simulink model "Evaluate_inertia_and_damping"  (R2016b)
settings: Solver=ode1  StartTime=0.0  StopTime=pre_time + s_t  FixedStep=T_sample  MinStep=1e-4  RelTol=1e-3
undefined symbols (not defined in the file): Activator, pre_time, selector
libraries: qbmove_library x2, QB_pacer_lib x1
settings Model: Creator=Franco  LastModifiedBy=Franco
settings DataIOCC: LimitDataPoints=on  SaveFormat=Array  SignalLoggingSaveFormat=ModelDataLogs
settings OptimizationCC: ExpressionDepthLimit=2147483647  EfficientMapNaN2IntZero=off  LifeSpan=inf
settings DebuggingCC: UnderspecifiedInitializationDetection=Classic  MergeDetectMultiDrivingBlocksExec=none  SolverPrmCheckMsg=warning  FcnCallInpInsideContextMsg=warning  AllowSymbolicDim=off  StateNameClashWarn=warning  SFUnexpectedBacktrackingDiag=warning  SFNoUnconditionalDefaultTransitionDiag=warning  SFExecutionAtInitializationDiag=none
settings HardwareCC: ProdBitPerPointer=32  ProdBitPerSizeT=32  ProdBitPerPtrDiffT=32  ProdLargestAtomicFloat=None  ProdIntDivRoundTo=Undefined  ProdEndianess=Unspecified  ProdWordSize=32  ProdHWDeviceType=32-bit Generic  TargetBitPerPointer=64  TargetBitPerSizeT=64  TargetBitPerPtrDiffT=64  TargetLongLongMode=on  TargetIntDivRoundTo=Zero  TargetEndianess=LittleEndian  TargetWordSize=64  TargetHWDeviceType=MATLAB Host  ProdEqTarget=off
settings ModelReferenceCC: PropagateSignalLabelsOutOfModel=off
settings CodeAppCC: MaxIdLength=128
settings GRTTargetCC: TargetLangStandard=C89/C90 (ANSI)  GeneratePreprocessorConditionals=Disable all  CombineOutputUpdateFcns=off  GRTInterface=on
settings ConfigComp: CovMetricSettings=dw  CovHtmlReporting=on  CovSaveCumulativeToWorkspaceVar=on  CovSaveSingleToWorkspaceVar=on  CovExternalEMLEnable=off  CovSFcnEnable=off
settings ConfigurationSet: Description=SimMechanics 2G

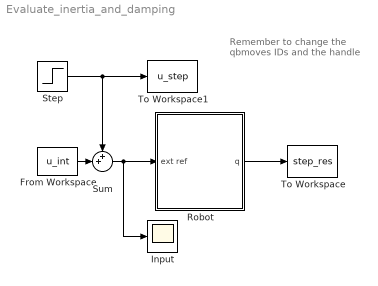
== system Evaluate_inertia_and_damping ==
  note: Remember to change the qbmoves IDs and the handle
  From Workspace : FromWorkspace  VariableName=u_int  SampleTime=0  OutputAfterFinalValue=Setting to zero
  Input : Scope
  Robot : Subsystem
  Step : Step  Time=pre_time  After=selector  SampleTime=0
  Sum : Sum  Inputs=++|
  To Workspace : ToWorkspace  VariableName=step_res  SaveFormat=Structure With Time  SampleTime=-1
  To Workspace1 : ToWorkspace  VariableName=u_step  SaveFormat=Structure With Time  SampleTime=-1
  wires:
  From Workspace/1 -> Sum/2
  Sum/1 -> Robot/1("ext ref "), Input/1
  Step/1 -> Sum/1, To Workspace1/1
  Robot/1(q) -> To Workspace/1

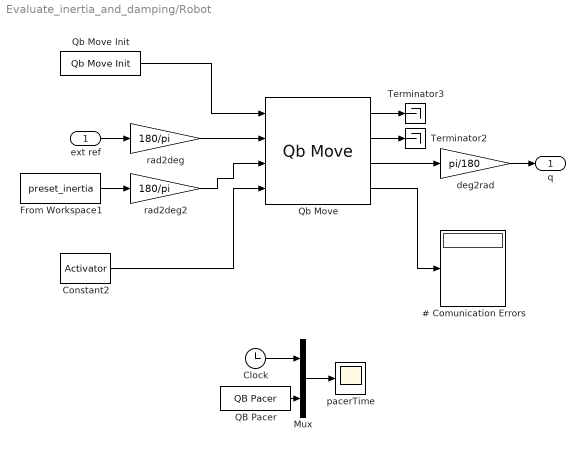
== system Evaluate_inertia_and_damping/Robot ==
  "ext ref " : Inport
  # Comunication Errors : Display
  Clock : Clock
  Constant2 : Constant  Value=Activator
  From Workspace1 : FromWorkspace  VariableName=preset_inertia  SampleTime=0  OutputAfterFinalValue=Setting to zero
  Mux : Mux  Inputs=2
  QB Pacer : QB_pacer_lib/QB Pacer  simTimePerRealTime=1
  Qb Move : qbmove_library/Qb Move  ID=[1 2 3 4 5 6]  ACTIVE_COMM_DIRECTIONS=Both  CONTROL_MODE=Equilibrium Position and Stiffness Preset  DAISY_CHAINING=off  MAX_ANG=0  SW_LIMIT=inf  OFFSET=0  ACTIVATE=off  WDT=0.0  UNIT=Degrees
  Qb Move Init : qbmove_library/Qb Move Init  NUMBER_OF_COM='COM7'  BAUD_RATE_COM=2000000
  Terminator2 : Terminator
  Terminator3 : Terminator
  deg2rad : Gain  Gain=pi/180
  pacerTime : Scope
  rad2deg : Gain  Gain=180/pi
  rad2deg2 : Gain  Gain=180/pi
  q : Outport
  wires:
  deg2rad/1 -> q/1
  "ext ref "/1 -> rad2deg/1
  From Workspace1/1 -> rad2deg2/1
  QB Pacer/1 -> Mux/2
  Clock/1 -> Mux/1
  Qb Move Init/1 -> Qb Move/1
  Mux/1 -> pacerTime/1
  Qb Move/1 -> Terminator3/1
  Qb Move/2 -> Terminator2/1
  Qb Move/3 -> deg2rad/1
  rad2deg/1 -> Qb Move/2
  Qb Move/4 -> # Comunication Errors/1
  rad2deg2/1 -> Qb Move/3
  Constant2/1 -> Qb Move/4
